simulink model "crude_filtering"  (R2018a)
settings: Solver=VariableStepAuto  StartTime=0.0  StopTime=10.0  RelTol=1e-3
settings Model: Creator=tlasi  LastModifiedBy=tlasi

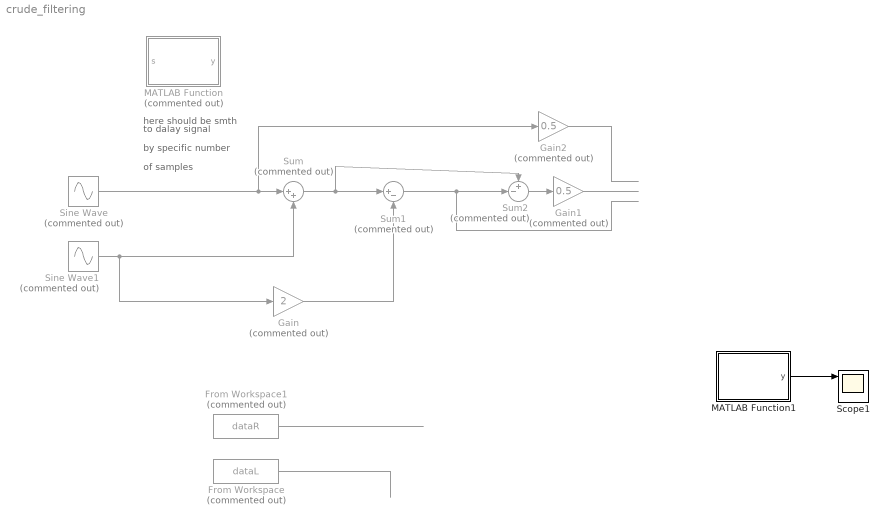
== system crude_filtering ==
  note: to dalay signal
  note: of samples
  note: by specific number
  note: here should be smth
  From Workspace : FromWorkspace  Commented=on  VariableName=dataL
  From Workspace1 : FromWorkspace  Commented=on  VariableName=dataR  OutDataTypeStr=fixdt(1,16,0)  SampleTime=1/48000
  Gain : Gain  Commented=on  Gain=2
  Gain1 : Gain  Commented=on  Gain=0.5
  Gain2 : Gain  Commented=on  Gain=0.5
  MATLAB Function : MATLAB Function  Commented=on  TreatAsAtomicUnit=on
  MATLAB Function1 : MATLAB Function  TreatAsAtomicUnit=on
  Scope1 : Scope  NumInputPorts=3
  Sine Wave : Sin  Commented=on  SampleTime=0
  Sine Wave1 : Sin  Commented=on  Phase=0.5  SampleTime=0
  Sum : Sum  Commented=on  Inputs=|++
  Sum1 : Sum  Commented=on  Inputs=|+-
  Sum2 : Sum  Commented=on  Inputs=+-|
  wires:
  Sine Wave1/1 -> Gain/1, Sum/2
  Sine Wave/1 -> Gain2/1, Sum/1
  Sum/1 -> Sum2/1, Sum1/1
  Gain/1 -> Sum1/2
  Sum1/1 -> Sum2/2
  Sum2/1 -> Gain1/1
  Gain1/1 -> ?
  Gain2/1 -> ?
  From Workspace1/1 -> ?
  From Workspace/1 -> ?
  MATLAB Function1/1(y) -> Scope1/1

== matlab function crude_filtering/MATLAB Function1 ==
  data: y output
function y = fcn()
Fs=48000;
[y,Fs] = audioread('LeftMicSampleCenter.flac');

== matlab function crude_filtering/MATLAB Function ==
  data: s input; y output
function y = fcn(s)
s = zeros(size(x));
if shift >0
	s(shift+1:end) = x(1:end-shift);
elseif shift <0
	s(1:end+shift) = x(-shift+1:end);
end
y = s;
